simulink model "close_loop_system_avance_phase_pi"  (Simulink 7.7)
settings: Solver=ode45  StartTime=0.0  StopTime=10.0  RelTol=1e-3
values from neighbouring files (symbols this model uses):
  a = (1+sind(PhD))/(1-sind(PhD))    [BE7_trame.m]
  Jt = 0.002    [BE7_trame.m]
  K_av = aK_av/a    [BE7_trame.m]
  Kci = 1    [BE7_trame.m]
  Kcp = 1    [BE7_trame.m]
  Kcv = 0.0314    [BE7_trame.m]
  Ke = 0.2    [BE7_trame.m]
  Kg = 0.2    [BE7_trame.m]
  Le = 0.002    [BE7_trame.m]
  N = 300    [BE7_trame.m]
  Re = 2    [BE7_trame.m]
  T_av = 1/(Wc*sqrt(a))    [BE7_trame.m]
  T_pi = 10/W_pi    [BE7_trame.m]
libraries: simulink x2
settings Model: Creator=Anthony  LastModifiedBy=Anthony

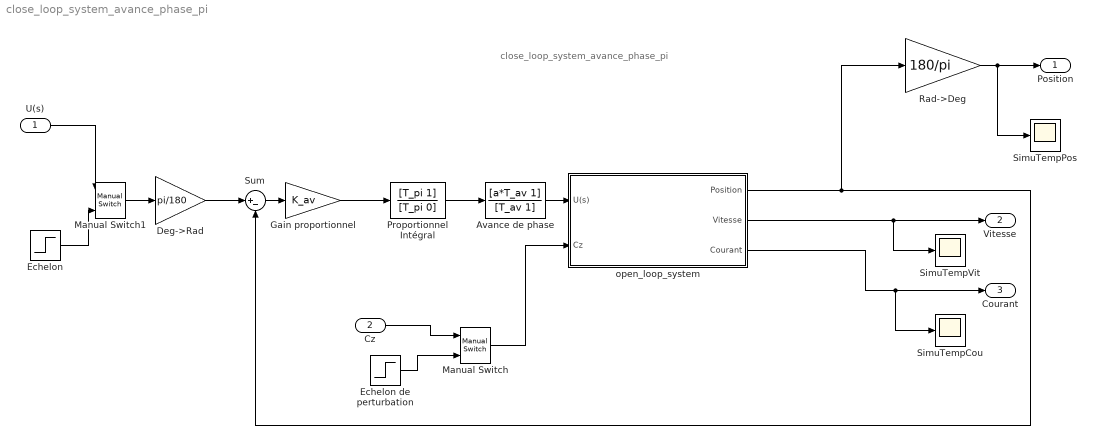
== system close_loop_system_avance_phase_pi ==
  note: close_loop_system_avance_phase_pi
  U(s) : Inport
  Cz : Inport  Port=2
  Avance de phase : TransferFcn  Numerator=[a*T_av 1]  Denominator=[T_av 1]
  Deg->Rad : Gain  Gain=pi/180
  Echelon : Step  Time=0  After=100  SampleTime=0
  "Echelon de perturbation " : Step  Time=5  After=5  SampleTime=0
  Gain proportionnel : Gain  Gain=K_av
  Manual Switch : simulink/Signal Routing/Manual Switch  SystemSampleTime=-1  sw=0  action=0  varsize=off
  Manual Switch1 : simulink/Signal Routing/Manual Switch  SystemSampleTime=-1  sw=0  action=0  varsize=off
  Proportionnel Intégral : TransferFcn  Numerator=[T_pi 1]  Denominator=[T_pi 0]
  Rad->Deg : Gain  Gain=180/pi
  SimuTempCou : Scope
      settings: SaveName=ScopeData2
  SimuTempPos : Scope
  SimuTempVit : Scope
  Sum : Sum  Inputs=|+-
  "open_loop_system " : Subsystem
  Position : Outport
  Vitesse : Outport  Port=2
  Courant : Outport  Port=3
  wires:
  "open_loop_system "/1(Position) -> Sum/2, Rad->Deg/1
  "open_loop_system "/3(Courant) -> SimuTempCou/1, Courant/1
  Sum/1 -> Gain proportionnel/1
  Gain proportionnel/1 -> Proportionnel Intégral/1
  Manual Switch1/1 -> Deg->Rad/1
  U(s)/1 -> Manual Switch1/1
  Echelon/1 -> Manual Switch1/2
  Avance de phase/1 -> "open_loop_system "/1(U(s))
  Cz/1 -> Manual Switch/1
  Manual Switch/1 -> "open_loop_system "/2(Cz)
  "Echelon de perturbation "/1 -> Manual Switch/2
  "open_loop_system "/2(Vitesse) -> SimuTempVit/1, Vitesse/1
  Rad->Deg/1 -> SimuTempPos/1, Position/1
  Deg->Rad/1 -> Sum/1
  Proportionnel Intégral/1 -> Avance de phase/1

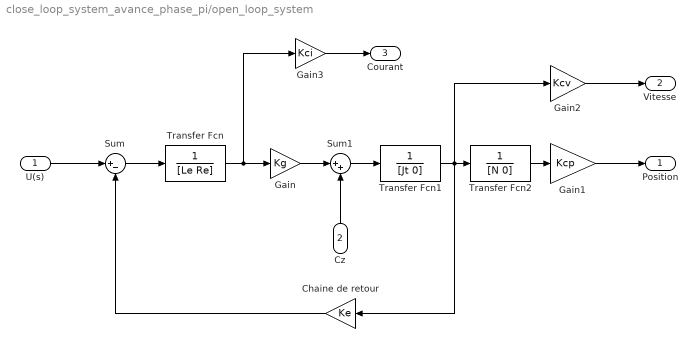
== system close_loop_system_avance_phase_pi/open_loop_system  ==
  U(s) : Inport
  Cz : Inport  Port=2
  Chaine de retour : Gain  Gain=Ke
  Gain : Gain  Gain=Kg
  Gain1 : Gain  Gain=Kcp
  Gain2 : Gain  Gain=Kcv
  Gain3 : Gain  Gain=Kci
  Sum : Sum  Inputs=|+-
  Sum1 : Sum  Inputs=|++
  Transfer Fcn : TransferFcn  Denominator=[Le Re]
  Transfer Fcn1 : TransferFcn  Denominator=[Jt 0]
  Transfer Fcn2 : TransferFcn  Denominator=[N 0]
  Position : Outport
  Vitesse : Outport  Port=2
  Courant : Outport  Port=3
  wires:
  Gain1/1 -> Position/1
  Gain3/1 -> Courant/1
  Gain2/1 -> Vitesse/1
  Cz/1 -> Sum1/2
  U(s)/1 -> Sum/1
  Transfer Fcn2/1 -> Gain1/1
  Transfer Fcn1/1 -> Chaine de retour/1, Transfer Fcn2/1, Gain2/1
  Transfer Fcn/1 -> Gain/1, Gain3/1
  Sum/1 -> Transfer Fcn/1
  Sum1/1 -> Transfer Fcn1/1
  Gain/1 -> Sum1/1
  Chaine de retour/1 -> Sum/2
